simulink model "bf_ranger_indi_continu_simutemp"  (R2021a)
settings: Solver=VariableStepAuto  StartTime=0.0  StopTime=10  RelTol=1e-3
values from neighbouring files (symbols this model uses):
  Ah3 = blkdiag(Ah3, Ahc)    [ranger_sim.m]
  Ah7 = blkdiag(Ah7, Ahc)    [ranger_sim.m]
  Amc = d2c(Amd,'tustin')    [ranger_sim.m]
  Asc = d2c(Asd,'tustin')    [ranger_sim.m]
  Bh3 = blkdiag(Bh3, Bhc)    [ranger_sim.m]
  Bh7 = blkdiag(Bh7, Bhc)    [ranger_sim.m]
  Ch3 = blkdiag(Ch3, Chc)    [ranger_sim.m]
  Ch7 = blkdiag(Ch7, Chc)    [ranger_sim.m]
  Dh3 = blkdiag(Dh3, Dhc)    [ranger_sim.m]
  Dh7 = blkdiag(Dh7, Dhc)    [ranger_sim.m]
  G = [-10.67  10.67  0     0     0     0 0 ... (first row only)    [ranger_sim.m]
  G_inv = pinv(G)    [ranger_sim.m]
  G_thrust = [0 0 0 0 0 0 0 ... (first row only)    [ranger_sim.m]
  Kd = [10; 18; 18]    [ranger_sim.m]
  Kp = [4.1089; 4.7304; 7.36]    [ranger_sim.m]
settings Model: Creator=AutomZ2-RG02B04  LastModifiedBy=AutomZ2-RG02A02
settings SolverCC: AlgebraicLoopSolver=TrustRegion

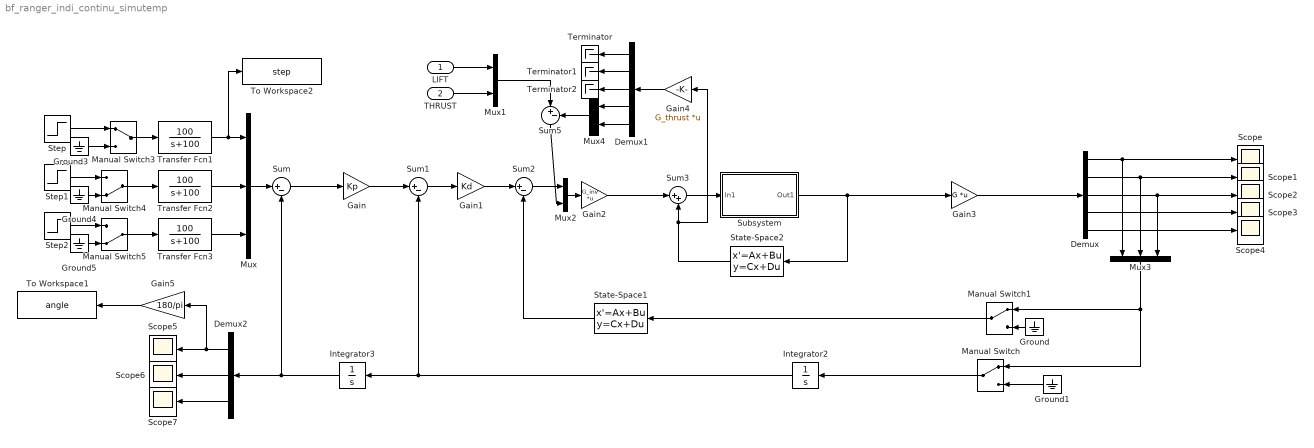
== system bf_ranger_indi_continu_simutemp ==
  LIFT : Inport
  THRUST : Inport  Port=2
  Demux : Demux  Outputs=5
  Demux1 : Demux  Outputs=5
  Demux2 : Demux  Outputs=3
  Gain : Gain  Gain=Kp
  Gain1 : Gain  Gain=Kd
  Gain2 : Gain  Gain=G_inv  Multiplication=Matrix(K*u)
  Gain3 : Gain  Gain=G  Multiplication=Matrix(K*u)
  Gain4 : Gain  Gain=G_thrust  Multiplication=Matrix(K*u)
  Gain5 : Gain  Gain=180/pi
  Ground{,1,3..5} (5 alike) : Ground
  Integrator2 : Integrator
  Integrator3 : Integrator
  Manual Switch : ManualSwitch
  Manual Switch1 : ManualSwitch
  Manual Switch3 : ManualSwitch
  Manual Switch4 : ManualSwitch  CurrentSetting=0
  Manual Switch5 : ManualSwitch  CurrentSetting=0
  Mux : Mux  Inputs=3
  Mux1 : Mux  Inputs=2
  Mux2 : Mux  Inputs=[3 2]
  Mux3 : Mux  Inputs=3
  Mux4 : Mux  Inputs=2
  Scope{,1..7} (8 alike) : Scope
  State-Space1 : StateSpace  A=Ah3  B=Bh3  C=Ch3  D=Dh3  InitialCondition=0
  State-Space2 : StateSpace  A=Ah7  B=Bh7  C=Ch7  D=Dh7  InitialCondition=0
  Step : Step  Time=0  After=20*pi/180  SampleTime=0
  Step1 : Step  Time=0  After=20*pi/180  SampleTime=0
  Step2 : Step  Time=0  After=20*pi/180  SampleTime=0
  Subsystem : Subsystem
  Sum{,1..2,5} (4 alike) : Sum  Inputs=|+-
  Sum3 : Sum  Inputs=|++
  Terminator : Terminator
  Terminator1 : Terminator
  Terminator2 : Terminator
  To Workspace1 : ToWorkspace  VariableName=angle  SaveFormat=Structure With Time  SampleTime=0.002
  To Workspace2 : ToWorkspace  VariableName=step  SaveFormat=Structure With Time  SampleTime=0.002
  Transfer Fcn1 : TransferFcn  Numerator=[100]  Denominator=[1 100]
  Transfer Fcn2 : TransferFcn  Numerator=[100]  Denominator=[1 100]
  Transfer Fcn3 : TransferFcn  Numerator=[100]  Denominator=[1 100]
  wires:
  Sum/1 -> Gain/1
  Gain/1 -> Sum1/1
  Sum1/1 -> Gain1/1
  Gain1/1 -> Sum2/1
  Sum2/1 -> Mux2/1
  Gain2/1 -> Sum3/1
  Mux1/1 -> Sum5/1
  Mux2/1 -> Gain2/1
  Sum3/1 -> Subsystem/1(In1)
  Mux/1 -> Sum/1
  LIFT/1 -> Mux1/1
  THRUST/1 -> Mux1/2
  Sum5/1 -> Mux2/2
  Demux/1 -> Scope/1, Mux3/1
  Demux/2 -> Mux3/2, Scope1/1
  Demux/3 -> Scope2/1, Mux3/3
  Demux/4 -> Scope3/1
  Demux/5 -> Scope4/1
  Gain4/1 -> Demux1/1
  Mux4/1 -> Sum5/2
  Demux1/4 -> Mux4/1
  Demux1/5 -> Mux4/2
  Demux1/1 -> Terminator/1
  Demux1/2 -> Terminator1/1
  Demux1/3 -> Terminator2/1
  Gain3/1 -> Demux/1
  Integrator2/1 -> Sum1/2, Integrator3/1
  State-Space2/1 -> Gain4/1, Sum3/2
  State-Space1/1 -> Sum2/2
  Mux3/1 -> Manual Switch/1, Manual Switch1/1
  Manual Switch1/1 -> State-Space1/1
  Ground/1 -> Manual Switch1/2
  Manual Switch/1 -> Integrator2/1
  Ground1/1 -> Manual Switch/2
  Subsystem/1(Out1) -> Gain3/1, State-Space2/1
  Step/1 -> Manual Switch3/1
  Manual Switch3/1 -> Transfer Fcn1/1
  Ground3/1 -> Manual Switch3/2
  Ground4/1 -> Manual Switch4/2
  Manual Switch4/1 -> Transfer Fcn2/1
  Step1/1 -> Manual Switch4/1
  Transfer Fcn2/1 -> Mux/2
  Step2/1 -> Manual Switch5/1
  Manual Switch5/1 -> Transfer Fcn3/1
  Ground5/1 -> Manual Switch5/2
  Transfer Fcn3/1 -> Mux/3
  Transfer Fcn1/1 -> To Workspace2/1, Mux/1
  Demux2/2 -> Scope6/1
  Integrator3/1 -> Demux2/1, Sum/2
  Demux2/1 -> Gain5/1, Scope5/1
  Demux2/3 -> Scope7/1
  Gain5/1 -> To Workspace1/1

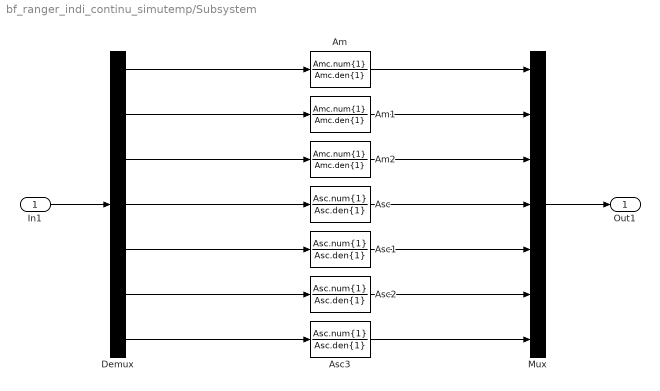
== system bf_ranger_indi_continu_simutemp/Subsystem ==
  In1 : Inport
  Am : TransferFcn  Numerator=Amc.num{1}  Denominator=Amc.den{1}
  Am1 : TransferFcn  Numerator=Amc.num{1}  Denominator=Amc.den{1}
  Am2 : TransferFcn  Numerator=Amc.num{1}  Denominator=Amc.den{1}
  Asc{,1..3} (4 alike) : TransferFcn  Numerator=Asc.num{1}  Denominator=Asc.den{1}
  Demux : Demux  Outputs=7
  Mux : Mux  Inputs=7
  Out1 : Outport
  wires:
  Demux/5 -> Asc1/1
  Asc/1 -> Mux/4
  Demux/4 -> Asc/1
  Asc1/1 -> Mux/5
  Asc2/1 -> Mux/6
  Demux/6 -> Asc2/1
  Asc3/1 -> Mux/7
  Demux/7 -> Asc3/1
  In1/1 -> Demux/1
  Mux/1 -> Out1/1
  Demux/1 -> Am/1
  Am/1 -> Mux/1
  Am1/1 -> Mux/2
  Demux/2 -> Am1/1
  Am2/1 -> Mux/3
  Demux/3 -> Am2/1
